simulink subsystem "scenario_403stretch_short"  (R2022b)
settings: Solver=VariableStepAuto  StartTime=0.0  StopTime=10.0  RelTol=1e-3
undefined symbols (not defined in the file or in its folder): driving
libraries: drivingscenarioandsensors x9
(part 1 of 3)
settings Model: Creator=smryk  LastModifiedBy=smryk

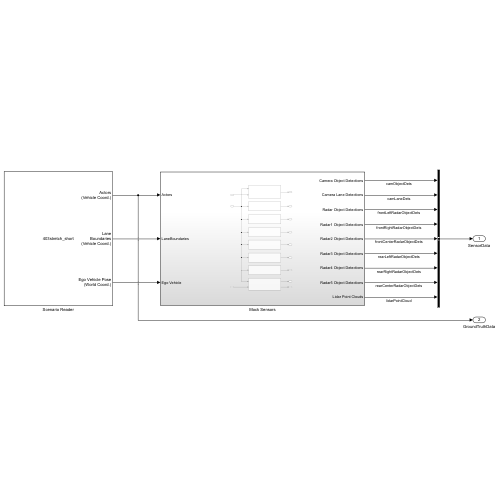
[thumbnail: Simulink's stored preview of the top-level diagram]
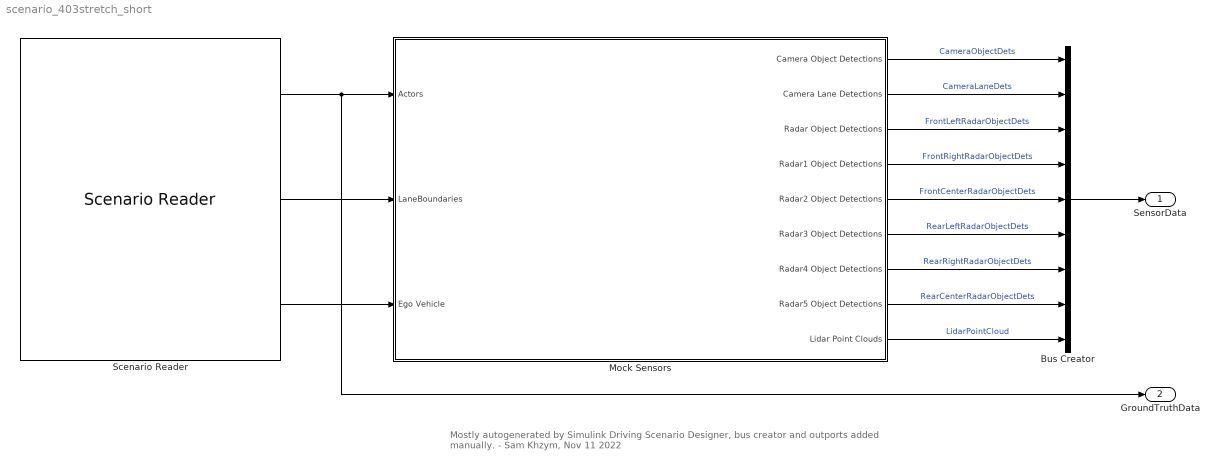
== system scenario_403stretch_short ==
  note: Mostly autogenerated by Simulink Driving Scenario Designer, bus creator and outports added manually. - Sam Khzym, Nov 11 2022
  Bus Creator : BusCreator  Inputs=9  OutDataTypeStr=Bus: SensorData
  Mock Sensors : Subsystem
  Scenario Reader : drivingscenarioandsensors/Scenario Reader  ScenarioSource=From file  ScenarioFileName=C:\Users\smryk\Desktop\EcoCAR\EcoCAR EV\CAVs\Software\test-environment\scenarios\403stretch_short.mat  ScenarioVariableName=scenario  OutputCoordinateSystem=Vehicle coordinates  EgoVehicleSource=Scenario  EgoVehicleActorID=1  OrientVehiclesOnRoad=off  OutputEgoVehiclePose=on  OutputEgoVehicleState=off  SampleTime=0.1  LaneBoundaryOutput=Ego vehicle lane boundaries  LaneBoundaryDistance=linspace(-100, 100, 101)  LaneBoundaryLocation=Center of lane markings  BusNameSource=Auto  BusName=BusActors  BusNumActorsSource=Scenario  BusNumActors=100  BusName2Source=Auto  BusName2=BusLaneBoundaries  BusNumLaneBoundariesSource=Scenario  BusNumLaneBoundaries=10  BusName3Source=Auto  BusName3=BusEgoActor  BusName4Source=Auto  BusName4=BusEgoState  ShowCoordinateLabels=on  SimulateUsing=Interpreted execution
  SensorData : Outport
  GroundTruthData : Outport  Port=2
  wires:
  Bus Creator/1 -> SensorData/1
  Scenario Reader/3 -> Mock Sensors/3(Ego Vehicle)
  Scenario Reader/2 -> Mock Sensors/2(LaneBoundaries)
  Scenario Reader/1 -> GroundTruthData/1, Mock Sensors/1(Actors)
  Mock Sensors/7(Radar4 Object Detections) -> Bus Creator/7  "RearRightRadarObjectDets"
  Mock Sensors/6(Radar3 Object Detections) -> Bus Creator/6  "RearLeftRadarObjectDets"
  Mock Sensors/5(Radar2 Object Detections) -> Bus Creator/5  "FrontCenterRadarObjectDets"
  Mock Sensors/3(Radar Object Detections) -> Bus Creator/3  "FrontLeftRadarObjectDets"
  Mock Sensors/4(Radar1 Object Detections) -> Bus Creator/4  "FrontRightRadarObjectDets"
  Mock Sensors/9(Lidar Point Clouds) -> Bus Creator/9  "LidarPointCloud"
  Mock Sensors/1(Camera Object Detections) -> Bus Creator/1  "CameraObjectDets"
  Mock Sensors/2(Camera Lane Detections) -> Bus Creator/2  "CameraLaneDets"
  Mock Sensors/8(Radar5 Object Detections) -> Bus Creator/8  "RearCenterRadarObjectDets"
